simulink model "second_order_system_TESTING_OPENLOOP_CLOSEDLOOP"  (R2023a)
settings: Solver=VariableStepAuto  StartTime=0.0  StopTime=10.0  RelTol=1e-3
settings Model: Creator=mazen  LastModifiedBy=mazen

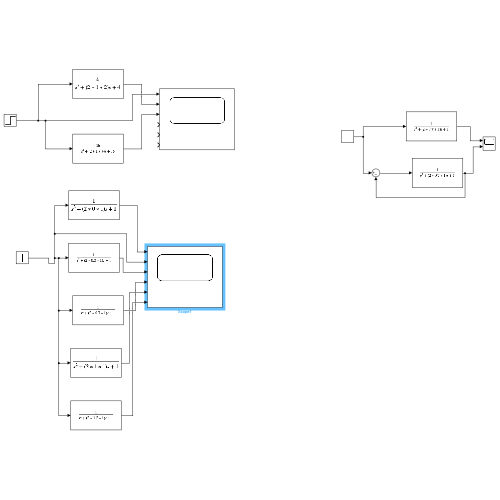
[thumbnail: Simulink's stored preview of the top-level diagram]
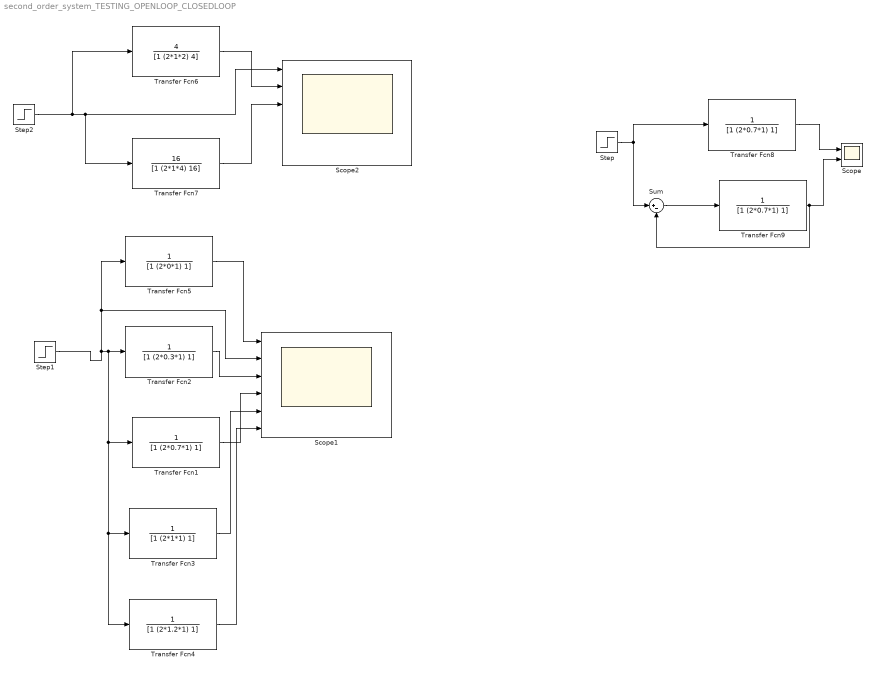
== system second_order_system_TESTING_OPENLOOP_CLOSEDLOOP ==
  Scope : Scope  NumInputPorts=2
  Scope1 : Scope  NumInputPorts=6
  Scope2 : Scope  NumInputPorts=6
  Step : Step  SampleTime=0
  Step1 : Step  SampleTime=0
  Step2 : Step  SampleTime=0
  Sum : Sum  Inputs=|+-
  Transfer Fcn1 : TransferFcn  Denominator=[1 (2*0.7*1) 1]
  Transfer Fcn2 : TransferFcn  Denominator=[1 (2*0.3*1) 1]
  Transfer Fcn3 : TransferFcn  Denominator=[1 (2*1*1) 1]
  Transfer Fcn4 : TransferFcn  Denominator=[1 (2*1.2*1) 1]
  Transfer Fcn5 : TransferFcn  Denominator=[1 (2*0*1) 1]
  Transfer Fcn6 : TransferFcn  Numerator=[4]  Denominator=[1 (2*1*2) 4]
  Transfer Fcn7 : TransferFcn  Numerator=[16]  Denominator=[1 (2*1*4) 16]
  Transfer Fcn8 : TransferFcn  Denominator=[1 (2*0.7*1) 1]
  Transfer Fcn9 : TransferFcn  Denominator=[1 (2*0.7*1) 1]
  wires:
  Transfer Fcn2/1 -> Scope1/3
  Step1/1 -> Transfer Fcn4/1, Transfer Fcn3/1, Transfer Fcn1/1, Transfer Fcn2/1, Transfer Fcn5/1, Scope1/2
  Transfer Fcn1/1 -> Scope1/4
  Transfer Fcn3/1 -> Scope1/5
  Transfer Fcn4/1 -> Scope1/6
  Transfer Fcn5/1 -> Scope1/1
  Transfer Fcn6/1 -> Scope2/2
  Transfer Fcn7/1 -> Scope2/3
  Step2/1 -> Transfer Fcn6/1, Transfer Fcn7/1, Scope2/1
  Sum/1 -> Transfer Fcn9/1
  Step/1 -> Sum/1, Transfer Fcn8/1
  Transfer Fcn8/1 -> Scope/1
  Transfer Fcn9/1 -> Sum/2, Scope/2
